simulink model "Soft_actuator_master_2021_experiments"  (R2020b)
settings: Solver=FixedStepAuto  StartTime=0.0  StopTime=inf  FixedStep=Ts  RelTol=1e-3  EnableMultiTasking=on
undefined symbols (not defined in the file): Pmax, Ts
libraries: arduinolib x7, simulink x1, dspfdesign x1
settings Model: SimulationMode=external  SILPILModeSetting=veronly  ExtModeTrigDuration=2  Creator=4D Lab  LastModifiedBy=Jakob Jansson
settings SolverCC: PositivePriorityOrder=on
settings OptimizationCC: EnhancedBackFolding=on  PassReuseOutputArgsAs=Individual arguments  ZeroExternalMemoryAtStartup=off  ZeroInternalMemoryAtStartup=off  MaxStackSize=64  OptimizeBlockOrder=speed  DifferentSizesBufferReuse=on  OptimizationCustomize=off  EfficientTunableParamExpr=on
settings DebuggingCC: ParameterTunabilityLossMsg=error
settings HardwareCC: ProdBitPerInt=16  ProdBitPerPointer=16  ProdBitPerSizeT=16  ProdBitPerPtrDiffT=16  ProdLargestAtomicFloat=None  ProdWordSize=8  ProdHWDeviceType=Atmel->AVR
settings RTWCC: Description=Embedded Coder  SystemTargetFile=ert.tlc  HardwareBoard=Arduino Mega 2560  TLCOptions="-aInlineSetEventsForThisBaseRateFcn=TLC_FALSE -aSuppressMultiTaskScheduler=TLC_FALSE   -aRateBasedStepFcn=1"  TemplateMakefile=ert_default_tmf  Toolchain=Arduino AVR  BuildConfiguration=Faster Runs
settings CodeAppCC: ForceParamTrailComments=on  IgnoreCustomStorageClasses=off  OperatorAnnotations=on  SimulinkDataObjDesc=on  SFDataObjDesc=on  InsertBlockDesc=on
settings ERTTargetCC: SupportContinuousTime=on  SupportVariableSizeSignals=on  ExtMode=on  ExtModeStaticAllocSize=2048  ExtModeMexArgs='127.0.0.1' 0 17725

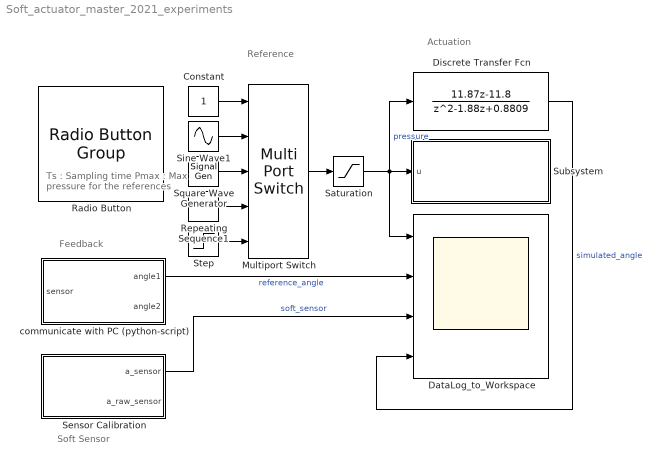
== system Soft_actuator_master_2021_experiments ==
  note: Reference
  note: Feedback
  note: Soft Sensor
  note: Actuation
  note: Ts : Sampling time
      | Pmax : Max pressure for the references
  Constant : Constant
  DataLog_to_Workspace : Scope  NumInputPorts=4
  Discrete Transfer Fcn : DiscreteTransferFcn  Numerator=[11.87 -11.8]  Denominator=[1 -1.88 0.8809]
  Multiport Switch : MultiPortSwitch  Inputs=4
  Radio Button : RadioButtonGroup  SelectedLabel=Sinewave  ButtonGroupName=Reference
      settings: Values={{'Sinewave', 'Squarewave', 'Ramp', 'Step'}, [1 2 3 4]}
  Repeating Sequence1 : simulink/Sources/Repeating Sequence  rep_seq_t=[0 4 6 10 12]  rep_seq_y=[0 0 Pmax Pmax 0]
  Saturation : Saturate  UpperLimit=6  LowerLimit=0
  Sensor Calibration : Subsystem
  Sine Wave1 : Sin  Amplitude=Pmax/2  Bias=Pmax/2  SampleTime=Ts
  Square Wave Generator : SignalGenerator  WaveForm=square  Amplitude=Pmax  Units=rad/sec
  Step : Step  After=Pmax  SampleTime=0
  Subsystem : Subsystem
  communicate with PC (python-script) : Subsystem
  wires:
  Discrete Transfer Fcn/1 -> DataLog_to_Workspace/4  "simulated_angle"
  Multiport Switch/1 -> Saturation/1
  Saturation/1 -> Discrete Transfer Fcn/1, DataLog_to_Workspace/1, Subsystem/1(u)  "pressure"
  Sensor Calibration/1(a_sensor) -> DataLog_to_Workspace/3  "soft_sensor"
  communicate with PC (python-script)/1(angle1) -> DataLog_to_Workspace/2  "reference_angle"
  Sine Wave1/1 -> Multiport Switch/2
  Constant/1 -> Multiport Switch/1
  Repeating Sequence1/1 -> Multiport Switch/4
  Square Wave Generator/1 -> Multiport Switch/3
  Step/1 -> Multiport Switch/5

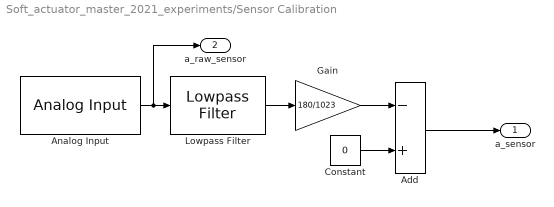
== system Soft_actuator_master_2021_experiments/Sensor Calibration ==
  Add : Sum  Inputs=-+
  Analog Input : arduinolib/Analog Input  pinNumber=4  ReadResultsOnly=off  ConversionTriggerSource=Software  ExternalTriggerType=uint32( 0 )  OutputDataType=uint16  EnableConversionCompleteNotify=off  EnableOuputStatus=off  SampleTime=Ts  blockPlatform=arduino
  Constant : Constant  Value=0
  Gain : Gain  Gain=180/1023
  Lowpass Filter : dspfdesign/Lowpass Filter  FilterType=FIR  DesignForMinimumOrder=on  FilterOrder=50  PassbandFrequency=8e3  StopbandFrequency=12e3  PassbandRipple=0.1  StopbandAttenuation=80  InheritSampleRate=off  SampleRate=44100  SimulateUsing=Interpreted execution  roundingMode=Floor  coeffsDataTypeStr=fixdt(1,16)
  a_sensor : Outport
  a_raw_sensor : Outport  Port=2
  wires:
  Gain/1 -> Add/1
  Constant/1 -> Add/2
  Analog Input/1 -> a_raw_sensor/1, Lowpass Filter/1
  Lowpass Filter/1 -> Gain/1
  Add/1 -> a_sensor/1

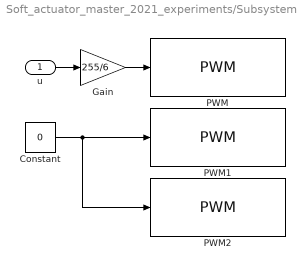
== system Soft_actuator_master_2021_experiments/Subsystem ==
  u : Inport
  Constant : Constant  Value=0
  Gain : Gain  Gain=255/6
  PWM : arduinolib/PWM  pinNumber=3  frequencyType=Default  desiredFrequency=490.2  achievableFrequency=490.2
  PWM1 : arduinolib/PWM  pinNumber=5  frequencyType=Default  desiredFrequency=490.2  achievableFrequency=490.2
  PWM2 : arduinolib/PWM  pinNumber=6  frequencyType=Default  desiredFrequency=490.2  achievableFrequency=490.2
  wires:
  Gain/1 -> PWM/1
  u/1 -> Gain/1
  Constant/1 -> PWM1/1, PWM2/1

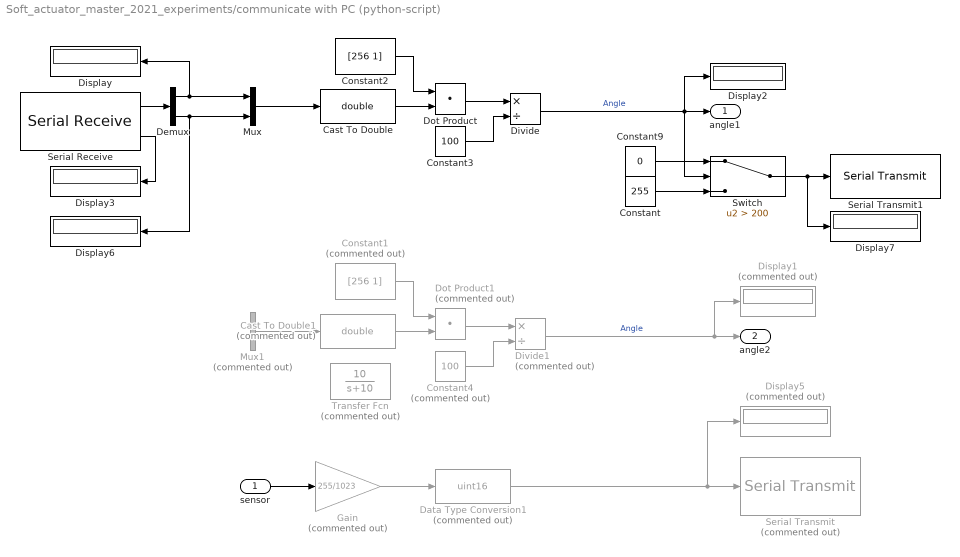
== system Soft_actuator_master_2021_experiments/communicate with PC (python-script) ==
  sensor : Inport
  Cast To Double : DataTypeConversion  OutDataTypeStr=double
  Cast To Double1 : DataTypeConversion  Commented=on  OutDataTypeStr=double
  Constant : Constant  Value=255
  Constant1 : Constant  Commented=on  Value=[256 1]
  Constant2 : Constant  Value=[256 1]
  Constant3 : Constant  Value=100
  Constant4 : Constant  Commented=on  Value=100
  Constant9 : Constant  Value=0
  Data Type Conversion1 : DataTypeConversion  Commented=on  OutDataTypeStr=uint16
  Demux : Demux  Outputs=2
  Display{,2..3,6..7} (5 alike) : Display
  Display1 : Display  Commented=on
  Display5 : Display  Commented=on
  Divide : Product  Inputs=*/
  Divide1 : Product  Commented=on  Inputs=*/
  Dot Product : DotProduct  InputSameDT=on  OutDataTypeStr=Inherit: Inherit via internal rule
  Dot Product1 : DotProduct  Commented=on  InputSameDT=on  OutDataTypeStr=Inherit: Inherit via internal rule
  Gain : Gain  Commented=on  Gain=255/1023  ParamDataTypeStr=uint16
  Mux : Mux  Inputs=2
  Mux1 : Mux  Commented=on  Inputs=2
  Serial Receive : arduinolib/Serial Receive  isARMArch=off  portNumber=1  DataType=uint8  Datalength=2  SampleTime=Ts  showOutStatus=on  blockPlatform=arduino
      settings: SourceProductBaseCode=ARDUINO
  Serial Transmit : arduinolib/Serial Transmit  Commented=on  portNumber=1  sendmode=println  sendformat=Decimal  floatprecision=2  blockPlatform=arduino
  Serial Transmit1 : arduinolib/Serial Transmit  portNumber=1  sendmode=write  sendformat=Decimal  floatprecision=2  blockPlatform=arduino
  Switch : Switch  Criteria=u2 > Threshold  Threshold=200
  Transfer Fcn : TransferFcn  Commented=on  Numerator=[10]  Denominator=[1 10]
  angle1 : Outport  VectorParamsAs1DForOutWhenUnconnected=off
  angle2 : Outport  Port=2  VectorParamsAs1DForOutWhenUnconnected=off
  wires:
  Constant3/1 -> Divide/2
  Cast To Double/1 -> Dot Product/2
  Constant2/1 -> Dot Product/1
  Dot Product/1 -> Divide/1
  Serial Receive/1 -> Demux/1
  Demux/1 -> Mux/1, Display/1
  Demux/2 -> Display6/1, Mux/2
  Dot Product1/1 -> Divide1/1
  Constant4/1 -> Divide1/2
  Cast To Double1/1 -> Dot Product1/2
  Constant1/1 -> Dot Product1/1
  Mux/1 -> Cast To Double/1
  Mux1/1 -> Cast To Double1/1
  Divide1/1 -> Display1/1, angle2/1  "Angle"
  Serial Receive/2 -> Display3/1
  Data Type Conversion1/1 -> Display5/1, Serial Transmit/1
  Gain/1 -> Data Type Conversion1/1
  sensor/1 -> Gain/1
  Divide/1 -> Switch/2, Display2/1, angle1/1  "Angle"
  Switch/1 -> Display7/1, Serial Transmit1/1
  Constant/1 -> Switch/3
  Constant9/1 -> Switch/1
